simulink library "xbsIndex_r3"  (Simulink 6.1)
PreLoadFcn:
  | xlmeta;
undefined symbols (not defined in the file or in its folder): sim_pause
libraries: xbsIndex_r3 x62, simulink x1
(part 4 of 4)

== system xbsIndex_r3/ System Generator ==
  2x System Clock : DiscretePulseGenerator  SampleTime=simulink_period
  Continuous Source : DiscretePulseGenerator  PulseType=Time based  Period=2*simulink_period  PulseWidth=50
  Terminator : Terminator
  Terminator1 : Terminator
  wires:
  2x System Clock/1 -> Terminator/1
  Continuous Source/1 -> Terminator1/1

== system xbsIndex_r3/Configurable Subsystem Manager ==
  2x System Clock : DiscretePulseGenerator
  Continuous Source : DiscretePulseGenerator  PulseType=Time based  PulseWidth=50
  Terminator : Terminator
  Terminator1 : Terminator
  wires:
  2x System Clock/1 -> Terminator/1
  Continuous Source/1 -> Terminator1/1

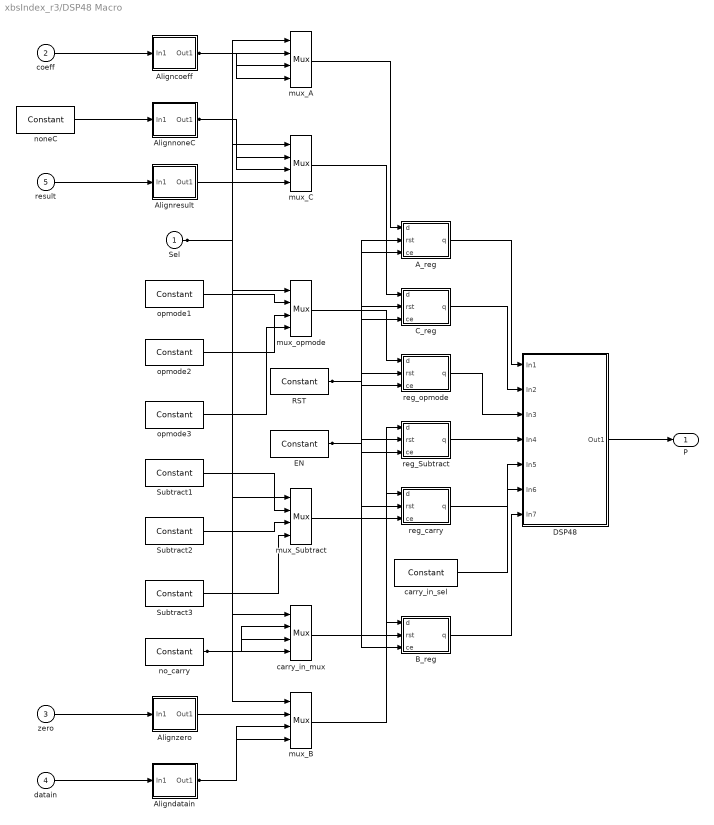
== system xbsIndex_r3/DSP48 Macro ==
  Sel : Inport  Port=1  LatchInput=off
  coeff : Inport  Port=2  LatchInput=off
  zero : Inport  Port=3  LatchInput=off
  datain : Inport  Port=4  LatchInput=off
  result : Inport  Port=5  LatchInput=off
  A_reg : Subsystem  mask{nreg=1, pnreg=1}
      mask prompts: nreg "Number of registers"; pnreg "Previous number of register"
      mask init:
      | [bg,fg] = xlcmap('XBlock',0);
      | iPos = get_param(gcb,'Position');
      | iWidth=iPos(3)-iPos(1); iHeight=iPos(4)-iPos(2);
      | iCx=iWidth/2;
      | iCy=iHeight/2;
      | [logoX, logoY] = xlogo(iPos);
      | str = sprintf('-%d',nreg);
      | sav_gcb = gcb;
      | set_param(sav_gcb,'linkstatus','none');
      | if (nreg ~= pnreg)
      |     sav_gcb  = gcb;
      |     regs     = find_system(sav_gcb, 'lookUnderMasks', 'all', 'masktype', 'Xilinx Register Block');
      |     terms    = find_system(sav_gcb, 'lookUnderMasks', 'all', 'BlockType', 'Terminator');
      |     inports  = find_system(sav_gcb, 'lookUnderMasks', 'all', 'BlockType', 'Inport');
      |     outports = find_system(sav_gcb, 'lookUnderMasks', 'all', 'BlockType', 'Outport');
      |       
      |     % delete all lines
      |     lines = get_param(sav_gcb, 'Lines');
      |     for i = 1:length(lines)
      |         delete_line(sav_gcb, lines(i,:).Points(1,:));
      |     end
      |       
      |     for i = 1:length(regs)
      |         delete_block(regs{i});
      |     end
      |     for i = 1:length(terms)
      |         delete_block(terms{i});
      |     end
      |     switch(nreg)
      |       case 0
      |           add_block('built-in/Terminator', [sav_gcb '/Terminator1'], 'position', [170   180   190   200]);
      |           add_block('built-in/Terminator', [sav_gcb '/Terminator2'], 'position', [240   195   260   215]);
      |           add_line(sav_gcb, 'd/1',   'q/1',           'autorouting', 'on');
      |           add_line(sav_gcb, 'rst/1', 'Terminator1/1', 'autorouting', 'on');
      |           add_line(sav_gcb, 'ce/1',  'Terminator2/1', 'autorouting', 'on');
      |       case 1
      |           add_block('xbsIndex_r3/Register', [sav_gcb '/Register1'], 'en', 'on', 'rst', 'on', 'position', [245   166   290   214]);
      |           add_line(sav_gcb, 'd/1',   'Register1/1',   'autorouting', 'on');
      |           add_line(sav_gcb, 'rst/1', 'Register1/2', 'autorouting', 'on');
      |           add_line(sav_gcb, 'ce/1',  'Register1/3', 'autorouting', 'on');
      |           add_line(sav_gcb, 'Register1/1', 'q/1',     'autorouting', 'on');
      |       case 2
      |           add_block('xbsIndex_r3/Register', [sav_gcb '/Register1'], 'en', 'on', 'rst', 'on', 'position', [245   166   290   214]);
      |           add_block('xbsIndex_r3/Register', [sav_gcb '/Register2'], 'en', 'on', 'rst', 'on', 'position', [385   181   430   229]);
      |           add_line(sav_gcb, 'd/1',   'Register1/1',   'autorouting', 'on');
      |           add_line(sav_gcb, 'rst/1', 'Register1/2', 'autorouting', 'on');
      |           add_line(sav_gcb, 'ce/1',  'Register1/3', 'autorouting', 'on');
      |           add_line(sav_gcb, 'Register1/1', 'Register2/1', 'autorouting', 'on');
      |           add_line(sav_gcb, 'rst/1', 'Register2/2', 'autorouting', 'on');
      |           add_line(sav_gcb, 'ce/1',  'Register2/3', 'autorouting', 'on');
      |           add_line(sav_gcb, 'Register2/1', 'q/1',   'autorouting', 'on');
      |      otherwise
      |           error('Illegal Mask Parameter to Register.  Allowed values are 0, 1, 2.');
      |     end
      |     set_param(sav_gcb, 'pnreg', int2str(nreg));
      | end
      mask Display:
      | patch([0 iWidth iWidth 0],[0 0 iHeight iHeight] , bg);
      | patch(logoX,logoY , fg);
      | text(iCx-6,iCy,'z');
      | text(iCx,iCy+4,str);
      | port_label('input',1,'d');
      | port_label('input',2,'rst');
      | port_label('input',3,'ce');
      | port_label('output',1,'q');
      | plot([0 0 iWidth iWidth 0], [0 iHeight iHeight 0 0]);
  Aligncoeff : Subsystem  mask{n_bits=18, bin_pt=11, arith_type=Signed  (2's comp), portwidth=18, dbl_ovrd=0}
      mask prompts: n_bits "Number of bits"; bin_pt "Binary Point"; arith_type "Arithmetic type"; portwidth "Port width"
      mask init:
      | this_gcb = gcb;
      | set_param(this_gcb,'linkstatus','none');
      | [bg,fg] = xlcmap('XBlock',dbl_ovrd);
      | iPos = get_param(gcb,'Position');
      | iWidth=iPos(3)-iPos(1); iHeight=iPos(4)-iPos(2);
      | iCx=iWidth/2;
      | iCy=iHeight/2;
      | [logoX, logoY] = xlogo(iPos);
      mask StyleString: edit,edit,popup(Signed  (2's comp)|Unsigned),edit,edit
      mask Display:
      | patch([0 iWidth iWidth 0],[0 0 iHeight iHeight] , bg);
      | patch(logoX,logoY , fg);
      | plot([0 0 iWidth iWidth 0], [0 iHeight iHeight 0 0]);
  Aligndatain : Subsystem  mask{n_bits=18, bin_pt=0, arith_type=Signed  (2's comp), portwidth=18, dbl_ovrd=0}
      mask prompts: n_bits "Number of bits"; bin_pt "Binary Point"; arith_type "Arithmetic type"; portwidth "Port width"
      mask init: same as xbsIndex_r3/DSP48 Macro/Aligncoeff
      mask StyleString: edit,edit,popup(Signed  (2's comp)|Unsigned),edit,edit
      mask Display:
      | patch([0 iWidth iWidth 0],[0 0 iHeight iHeight] , bg);
      | patch(logoX,logoY , fg);
      | plot([0 0 iWidth iWidth 0], [0 iHeight iHeight 0 0]);
  AlignnoneC : Subsystem  mask{n_bits=48, bin_pt=0, arith_type=Signed  (2's comp), portwidth=48, dbl_ovrd=0}
      mask prompts: n_bits "Number of bits"; bin_pt "Binary Point"; arith_type "Arithmetic type"; portwidth "Port width"
      mask init: same as xbsIndex_r3/DSP48 Macro/Aligncoeff
      mask StyleString: edit,edit,popup(Signed  (2's comp)|Unsigned),edit,edit
      mask Display:
      | patch([0 iWidth iWidth 0],[0 0 iHeight iHeight] , bg);
      | patch(logoX,logoY , fg);
      | plot([0 0 iWidth iWidth 0], [0 iHeight iHeight 0 0]);
  Alignresult : Subsystem  mask{n_bits=41, bin_pt=11, arith_type=Signed  (2's comp), portwidth=48, dbl_ovrd=0}
      mask prompts: n_bits "Number of bits"; bin_pt "Binary Point"; arith_type "Arithmetic type"; portwidth "Port width"
      mask init: same as xbsIndex_r3/DSP48 Macro/Aligncoeff
      mask StyleString: edit,edit,popup(Signed  (2's comp)|Unsigned),edit,edit
      mask Display:
      | patch([0 iWidth iWidth 0],[0 0 iHeight iHeight] , bg);
      | patch(logoX,logoY , fg);
      | plot([0 0 iWidth iWidth 0], [0 iHeight iHeight 0 0]);
  Alignzero : Subsystem  mask{n_bits=18, bin_pt=0, arith_type=Signed  (2's comp), portwidth=18, dbl_ovrd=0}
      mask prompts: n_bits "Number of bits"; bin_pt "Binary Point"; arith_type "Arithmetic type"; portwidth "Port width"
      mask init: same as xbsIndex_r3/DSP48 Macro/Aligncoeff
      mask StyleString: edit,edit,popup(Signed  (2's comp)|Unsigned),edit,edit
      mask Display:
      | patch([0 iWidth iWidth 0],[0 0 iHeight iHeight] , bg);
      | patch(logoX,logoY , fg);
      | plot([0 0 iWidth iWidth 0], [0 iHeight iHeight 0 0]);
  B_reg : Subsystem  mask{nreg=1, pnreg=1}
      mask prompts: nreg "Number of registers"; pnreg "Previous number of register"
      mask init: same as xbsIndex_r3/DSP48 Macro/A_reg
      mask Display:
      | patch([0 iWidth iWidth 0],[0 0 iHeight iHeight] , bg);
      | patch(logoX,logoY , fg);
      | text(iCx-6,iCy,'z');
      | text(iCx,iCy+4,str);
      | port_label('input',1,'d');
      | port_label('input',2,'rst');
      | port_label('input',3,'ce');
      | port_label('output',1,'q');
      | plot([0 0 iWidth iWidth 0], [0 iHeight iHeight 0 0]);
  C_reg : Subsystem  mask{nreg=2, pnreg=2}
      mask prompts: nreg "Number of registers"; pnreg "Previous number of register"
      mask init: same as xbsIndex_r3/DSP48 Macro/A_reg
      mask Display:
      | patch([0 iWidth iWidth 0],[0 0 iHeight iHeight] , bg);
      | patch(logoX,logoY , fg);
      | text(iCx-6,iCy,'z');
      | text(iCx,iCy+4,str);
      | port_label('input',1,'d');
      | port_label('input',2,'rst');
      | port_label('input',3,'ce');
      | port_label('output',1,'q');
      | plot([0 0 iWidth iWidth 0], [0 iHeight iHeight 0 0]);
  DSP48 : Subsystem  mask{dbl_ovrd=0}
      mask init:
      | this_gcb = gcb;
      | [bg,fg] = xlcmap('XBlock',dbl_ovrd);
      | iPos = get_param(gcb,'Position');
      | iWidth=iPos(3)-iPos(1); iHeight=iPos(4)-iPos(2);
      | iCx=iWidth/2;
      | iCy=iHeight/2;
      | [logoX, logoY] = xlogo(iPos);
      | set_param(this_gcb,'linkstatus','none');
      mask Display:
      | patch([0 iWidth iWidth 0],[0 0 iHeight iHeight] , bg);
      | patch(logoX,logoY , fg);
      | plot([0 0 iWidth iWidth 0], [0 iHeight iHeight 0 0]);
      | port_label('input',1,'A');
      | port_label('input',2,'C');
      | port_label('input',3,'Opmode');
      | port_label('input',4,'Subtract_sel');
      | port_label('input',5,'Carry');
      | port_label('input',6,'Carry_in_sel');
      | port_label('input',7,'B');
      | port_label('output',1,'P');
  EN : xbsIndex_r3/Constant  const=1  equ=P=C  arith_type=Boolean  n_bits=1  bin_pt=0  opselect=C  inp2=PCIN>>17  opr=+  inp1=P  carry=CIN  iostate=0  explicit_period=off  period=1  dbl_ovrd=off
  RST : xbsIndex_r3/Constant  const=0  equ=P=C  arith_type=Boolean  n_bits=1  bin_pt=0  opselect=C  inp2=PCIN>>17  opr=+  inp1=P  carry=CIN  iostate=0  explicit_period=off  period=1  dbl_ovrd=off
  Subtract1 : xbsIndex_r3/Constant  Tag=1  const=0  equ=P=C  arith_type=Boolean  n_bits=1  bin_pt=0  opselect=C  inp2=PCIN>>17  opr=+  inp1=P  carry=CIN  iostate=0  explicit_period=off  period=1  dbl_ovrd=off
  Subtract2 : xbsIndex_r3/Constant  Tag=2  const=0  equ=P=C  arith_type=Boolean  n_bits=1  bin_pt=0  opselect=C  inp2=PCIN>>17  opr=+  inp1=P  carry=CIN  iostate=0  explicit_period=off  period=1  dbl_ovrd=off
  Subtract3 : xbsIndex_r3/Constant  Tag=3  const=0  equ=P=C  arith_type=Boolean  n_bits=1  bin_pt=0  opselect=C  inp2=PCIN>>17  opr=+  inp1=P  carry=CIN  iostate=0  explicit_period=off  period=1  dbl_ovrd=off
  carry_in_mux : xbsIndex_r3/Mux  inputs=3  precision=Full  arith_type="Signed  (2's comp)"  n_bits=8  bin_pt=2  quantization=Truncate  overflow=Wrap  latency=0  explicit_period=off  period=1  en=off  dbl_ovrd=off  show_param=off  mux_type=off  use_rpm=off  gen_core=off
      settings: xl_area=[0, 0, 0, 0, 0, 0, 0]
  carry_in_sel : xbsIndex_r3/Constant  const=0  equ=P=C  arith_type=Unsigned  n_bits=2  bin_pt=0  opselect=C  inp2=PCIN>>17  opr=+  inp1=P  carry=CIN  iostate=0  explicit_period=off  period=1  dbl_ovrd=off
  mux_A : xbsIndex_r3/Mux  inputs=3  precision=User Defined  arith_type="Signed  (2's comp)"  n_bits=18  bin_pt=0  quantization=Truncate  overflow=Wrap  latency=0  explicit_period=off  period=1  en=off  dbl_ovrd=off  show_param=off  mux_type=off  use_rpm=off  gen_core=off
      settings: xl_area=[0, 0, 0, 0, 0, 0, 0]
  mux_B : xbsIndex_r3/Mux  inputs=3  precision=User Defined  arith_type="Signed  (2's comp)"  n_bits=18  bin_pt=0  quantization=Truncate  overflow=Wrap  latency=0  explicit_period=off  period=1  en=off  dbl_ovrd=off  show_param=off  mux_type=off  use_rpm=off  gen_core=off
      settings: xl_area=[0, 0, 0, 0, 0, 0, 0]
  mux_C : xbsIndex_r3/Mux  inputs=3  precision=User Defined  arith_type="Signed  (2's comp)"  n_bits=48  bin_pt=0  quantization=Truncate  overflow=Wrap  latency=0  explicit_period=off  period=1  en=off  dbl_ovrd=off  show_param=off  mux_type=off  use_rpm=off  gen_core=off
      settings: xl_area=[0, 0, 0, 0, 0, 0, 0]
  mux_Subtract : xbsIndex_r3/Mux  inputs=3  precision=Full  arith_type="Signed  (2's comp)"  n_bits=8  bin_pt=2  quantization=Truncate  overflow=Wrap  latency=0  explicit_period=off  period=1  en=off  dbl_ovrd=off  show_param=off  mux_type=off  use_rpm=off  gen_core=off
      settings: xl_area=[0, 0, 0, 0, 0, 0, 0]
  mux_opmode : xbsIndex_r3/Mux  inputs=3  precision=Full  arith_type="Signed  (2's comp)"  n_bits=8  bin_pt=2  quantization=Truncate  overflow=Wrap  latency=0  explicit_period=off  period=1  en=off  dbl_ovrd=off  show_param=off  mux_type=off  use_rpm=off  gen_core=off
      settings: xl_area=[0, 0, 0, 0, 0, 0, 0]
  no_carry : xbsIndex_r3/Constant  const=0  equ=P=C  arith_type=Unsigned  n_bits=1  bin_pt=0  opselect=C  inp2=PCIN>>17  opr=+  inp1=P  carry=CIN  iostate=0  explicit_period=off  period=1  dbl_ovrd=off
  noneC : xbsIndex_r3/Constant  const=0  equ=P=C  arith_type=Unsigned  n_bits=1  bin_pt=0  opselect=C  inp2=PCIN>>17  opr=+  inp1=P  carry=CIN  iostate=0  explicit_period=off  period=1  dbl_ovrd=off
  opmode1 : xbsIndex_r3/Constant  Tag=1  const=37  equ=P=C  arith_type=Unsigned  n_bits=7  bin_pt=0  opselect=C  inp2=PCIN>>17  opr=+  inp1=P  carry=CIN  iostate=0  explicit_period=off  period=1  dbl_ovrd=off
  opmode2 : xbsIndex_r3/Constant  Tag=2  const=5  equ=P=C  arith_type=Unsigned  n_bits=7  bin_pt=0  opselect=C  inp2=PCIN>>17  opr=+  inp1=P  carry=CIN  iostate=0  explicit_period=off  period=1  dbl_ovrd=off
  opmode3 : xbsIndex_r3/Constant  Tag=3  const=53  equ=P=C  arith_type=Unsigned  n_bits=7  bin_pt=0  opselect=C  inp2=PCIN>>17  opr=+  inp1=P  carry=CIN  iostate=0  explicit_period=off  period=1  dbl_ovrd=off
  reg_Subtract : Subsystem  mask{nreg=2, pnreg=2}
      mask prompts: nreg "Number of registers"; pnreg "Previous number of register"
      mask init: same as xbsIndex_r3/DSP48 Macro/A_reg
      mask Display:
      | patch([0 iWidth iWidth 0],[0 0 iHeight iHeight] , bg);
      | patch(logoX,logoY , fg);
      | text(iCx-6,iCy,'z');
      | text(iCx,iCy+4,str);
      | port_label('input',1,'d');
      | port_label('input',2,'rst');
      | port_label('input',3,'ce');
      | port_label('output',1,'q');
      | plot([0 0 iWidth iWidth 0], [0 iHeight iHeight 0 0]);
  reg_carry : Subsystem  mask{nreg=2, pnreg=2}
      mask prompts: nreg "Number of registers"; pnreg "Previous number of register"
      mask init: same as xbsIndex_r3/DSP48 Macro/A_reg
      mask Display:
      | patch([0 iWidth iWidth 0],[0 0 iHeight iHeight] , bg);
      | patch(logoX,logoY , fg);
      | text(iCx-6,iCy,'z');
      | text(iCx,iCy+4,str);
      | port_label('input',1,'d');
      | port_label('input',2,'rst');
      | port_label('input',3,'ce');
      | port_label('output',1,'q');
      | plot([0 0 iWidth iWidth 0], [0 iHeight iHeight 0 0]);
  reg_opmode : Subsystem  mask{nreg=2, pnreg=2}
      mask prompts: nreg "Number of registers"; pnreg "Previous number of register"
      mask init: same as xbsIndex_r3/DSP48 Macro/A_reg
      mask Display:
      | patch([0 iWidth iWidth 0],[0 0 iHeight iHeight] , bg);
      | patch(logoX,logoY , fg);
      | text(iCx-6,iCy,'z');
      | text(iCx,iCy+4,str);
      | port_label('input',1,'d');
      | port_label('input',2,'rst');
      | port_label('input',3,'ce');
      | port_label('output',1,'q');
      | plot([0 0 iWidth iWidth 0], [0 iHeight iHeight 0 0]);
  P : Outport
  wires:
  Sel/1 -> mux_C/1, mux_B/1, mux_A/1, carry_in_mux/1, mux_Subtract/1, mux_opmode/1
  RST/1 -> C_reg/2(rst), B_reg/2(rst), A_reg/2(rst), reg_carry/2(rst), reg_Subtract/2(rst), reg_opmode/2(rst)
  EN/1 -> C_reg/3(ce), B_reg/3(ce), A_reg/3(ce), reg_carry/3(ce), reg_Subtract/3(ce), reg_opmode/3(ce)
  no_carry/1 -> carry_in_mux/4, carry_in_mux/3, carry_in_mux/2
  Aligncoeff/1(Out1) -> mux_A/4, mux_A/3, mux_A/2
  Aligndatain/1(Out1) -> mux_B/4, mux_B/3
  AlignnoneC/1(Out1) -> mux_C/3, mux_C/2
  Alignresult/1(Out1) -> mux_C/4
  result/1 -> Alignresult/1(In1)
  noneC/1 -> AlignnoneC/1(In1)
  C_reg/1(q) -> DSP48/2(In2)
  mux_C/1 -> C_reg/1(d)
  datain/1 -> Aligndatain/1(In1)
  Alignzero/1(Out1) -> mux_B/2
  zero/1 -> Alignzero/1(In1)
  B_reg/1(q) -> DSP48/7(In7)
  mux_B/1 -> B_reg/1(d)
  coeff/1 -> Aligncoeff/1(In1)
  A_reg/1(q) -> DSP48/1(In1)
  mux_A/1 -> A_reg/1(d)
  reg_carry/1(q) -> DSP48/5(In5)
  carry_in_mux/1 -> reg_carry/1(d)
  carry_in_sel/1 -> DSP48/6(In6)
  Subtract3/1 -> mux_Subtract/4
  Subtract2/1 -> mux_Subtract/3
  Subtract1/1 -> mux_Subtract/2
  reg_Subtract/1(q) -> DSP48/4(In4)
  mux_Subtract/1 -> reg_Subtract/1(d)
  opmode3/1 -> mux_opmode/4
  opmode2/1 -> mux_opmode/3
  opmode1/1 -> mux_opmode/2
  reg_opmode/1(q) -> DSP48/3(In3)
  mux_opmode/1 -> reg_opmode/1(d)
  DSP48/1(Out1) -> P/1

== system xbsIndex_r3/Disregard Subsystem ==

== system xbsIndex_r3/FDATool ==
  Constant : Constant  Value=0  VectorParams1D=off  OutDataTypeMode=double
  Terminator : Terminator
  wires:
  Constant/1 -> Terminator/1

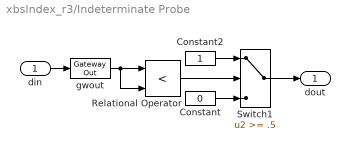
== system xbsIndex_r3/Indeterminate Probe ==
  din : Inport  Port=1  LatchInput=off
  Constant : Constant  Value=0
  Constant2 : Constant
  Relational Operator : RelationalOperator  Operator=<  InputSameDT=on
  Switch1 : Switch  Threshold=.5  SaturateOnIntegerOverflow=on  InputSameDT=on
  gwout : xbsIndex_r3/Gateway Out  output_type=Double  nbits=8  bin_pt=6  arith_type=Boolean  quantization=Truncate  overflow=Wrap  hdl_port=off  timing_constraint=None  locs_specified=off  LOCs={}  needs_fixed_name=off  show_param=off
      settings: xl_area=[0, 0, 0, 0, 0, 0, 0]
  dout : Outport
  wires:
  Switch1/1 -> dout/1
  Constant/1 -> Switch1/3
  Constant2/1 -> Switch1/1
  gwout/1 -> Relational Operator/2, Relational Operator/1
  Relational Operator/1 -> Switch1/2
  din/1 -> gwout/1

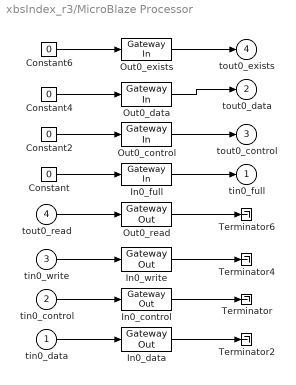
== system xbsIndex_r3/MicroBlaze Processor ==
  tin0_data : Inport  Tag=in0  Port=1  LatchInput=off
  tin0_control : Inport  Tag=in0  Port=2  LatchInput=off
  tin0_write : Inport  Tag=in0  Port=3  LatchInput=off
  tout0_read : Inport  Tag=out0  Port=4  LatchInput=off
  Constant{,2,4,6} (4 alike) : Constant  Value=0
  In0_control : xbsIndex_r3/Gateway Out  output_type=Double  nbits=8  bin_pt=6  arith_type=Boolean  quantization=Truncate  overflow=Wrap  hdl_port=on  timing_constraint=None  locs_specified=off  LOCs={}  needs_fixed_name=off  show_param=off
      settings: xl_area=[0, 0, 0, 0, 0, 0, 0]
  In0_data : xbsIndex_r3/Gateway Out  output_type=Double  nbits=8  bin_pt=6  arith_type=Boolean  quantization=Truncate  overflow=Wrap  hdl_port=on  timing_constraint=None  locs_specified=off  LOCs={}  needs_fixed_name=off  show_param=off
      settings: xl_area=[0, 0, 0, 0, 0, 0, 0]
  In0_full : xbsIndex_r3/Gateway In  arith_type=Unsigned  n_bits=1  bin_pt=0  quantization=Truncate  overflow=Wrap  period=1  timing_constraint=None  locs_specified=off  LOCs={}  needs_fixed_name=off  dbl_ovrd=off  show_param=off
      settings: xl_area=[0, 0, 0, 0, 0, 0, 0]
  In0_write : xbsIndex_r3/Gateway Out  output_type=Double  nbits=8  bin_pt=6  arith_type=Boolean  quantization=Truncate  overflow=Wrap  hdl_port=on  timing_constraint=None  locs_specified=off  LOCs={}  needs_fixed_name=off  show_param=off
      settings: xl_area=[0, 0, 0, 0, 0, 0, 0]
  Out0_control : xbsIndex_r3/Gateway In  arith_type=Unsigned  n_bits=1  bin_pt=0  quantization=Truncate  overflow=Wrap  period=1  timing_constraint=None  locs_specified=off  LOCs={}  needs_fixed_name=off  dbl_ovrd=off  show_param=off
      settings: xl_area=[0, 0, 0, 0, 0, 0, 0]
  Out0_data : xbsIndex_r3/Gateway In  arith_type=Unsigned  n_bits=32  bin_pt=0  quantization=Truncate  overflow=Wrap  period=1  timing_constraint=None  locs_specified=off  LOCs={}  needs_fixed_name=off  dbl_ovrd=off  show_param=off
      settings: xl_area=[0, 0, 0, 0, 0, 0, 0]
  Out0_exists : xbsIndex_r3/Gateway In  arith_type=Unsigned  n_bits=1  bin_pt=0  quantization=Truncate  overflow=Wrap  period=1  timing_constraint=None  locs_specified=off  LOCs={}  needs_fixed_name=off  dbl_ovrd=off  show_param=off
      settings: xl_area=[0, 0, 0, 0, 0, 0, 0]
  Out0_read : xbsIndex_r3/Gateway Out  output_type=Double  nbits=8  bin_pt=6  arith_type=Boolean  quantization=Truncate  overflow=Wrap  hdl_port=on  timing_constraint=None  locs_specified=off  LOCs={}  needs_fixed_name=off  show_param=off
      settings: xl_area=[0, 0, 0, 0, 0, 0, 0]
  Terminator{,2,4,6} (4 alike) : Terminator
  tin0_full : Outport  Tag=in0
  tout0_data : Outport  Tag=out0  Port=2
  tout0_control : Outport  Tag=out0  Port=3
  tout0_exists : Outport  Tag=out0  Port=4
  wires:
  Out0_read/1 -> Terminator6/1
  Constant6/1 -> Out0_exists/1
  Constant4/1 -> Out0_data/1
  Constant2/1 -> Out0_control/1
  In0_write/1 -> Terminator4/1
  Constant/1 -> In0_full/1
  In0_data/1 -> Terminator2/1
  In0_control/1 -> Terminator/1
  Out0_exists/1 -> tout0_exists/1
  Out0_control/1 -> tout0_control/1
  Out0_data/1 -> tout0_data/1
  In0_full/1 -> tin0_full/1
  tout0_read/1 -> Out0_read/1
  tin0_write/1 -> In0_write/1
  tin0_control/1 -> In0_control/1
  tin0_data/1 -> In0_data/1

== system xbsIndex_r3/Multiple Subsystem Generator ==
  note: This is the Design Stitcher tool.
  Constant : Constant
  Terminator : Terminator
  wires:
  Constant/1 -> Terminator/1

== system xbsIndex_r3/Pause Simulation ==
  din : Inport  Port=1  LatchInput=off
  Gateway Out : xbsIndex_r3/Gateway Out  output_type=Double  nbits=8  bin_pt=6  arith_type=Boolean  quantization=Truncate  overflow=Wrap  hdl_port=on  timing_constraint=None  locs_specified=off  LOCs={}  needs_fixed_name=off  show_param=off
      settings: xl_area=[0, 0, 0, 0, 0, 0, 0]
  Pause  Simulation : MATLABFcn  Priority=1000  MATLABFcn=sim_pause(u)  OutputDimensions=0  Output1D=off
  wires:
  din/1 -> Gateway Out/1
  Gateway Out/1 -> Pause  Simulation/1

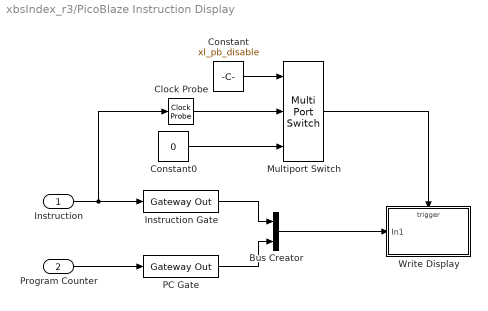
== system xbsIndex_r3/PicoBlaze Instruction Display ==
  Instruction : Inport  Port=1  LatchInput=off
  Program Counter : Inport  Port=2  LatchInput=off
  Bus Creator : BusCreator  DialogController=Simulink.DDGSource_Bus  Inputs=2
  Clock Probe : xbsIndex_r3/Clock Probe
  Constant : Constant  Value=xl_pb_disable
  Constant0 : Constant  Value=0
  Instruction Gate : xbsIndex_r3/Gateway Out  output_type=Double  nbits=8  bin_pt=6  arith_type=Boolean  quantization=Truncate  overflow=Wrap  hdl_port=off  timing_constraint=None  locs_specified=off  LOCs={}  needs_fixed_name=off  show_param=off
      settings: xl_area=[0, 0, 0, 0, 0, 0, 0]
  Multiport Switch : MultiPortSwitch  Inputs=2  zeroidx=on  SaturateOnIntegerOverflow=on
  PC Gate : xbsIndex_r3/Gateway Out  output_type=Double  nbits=8  bin_pt=6  arith_type=Boolean  quantization=Truncate  overflow=Wrap  hdl_port=off  timing_constraint=None  locs_specified=off  LOCs={}  needs_fixed_name=off  show_param=off
      settings: xl_area=[0, 0, 0, 0, 0, 0, 0]
  Write Display : Subsystem  mask{xl_pb_inst=LOAD sC, 12, xl_pb_pc=17, xl_pb_version=xl_pb_version}
      mask prompts: xl_pb_version "PicoBlaze Version"
  wires:
  Bus Creator/1 -> Write Display/1(In1)
  PC Gate/1 -> Bus Creator/2
  Instruction Gate/1 -> Bus Creator/1
  Program Counter/1 -> PC Gate/1
  Instruction/1 -> Instruction Gate/1, Clock Probe/1
  Constant/1 -> Multiport Switch/1
  Multiport Switch/1 -> Write Display/Trigger
  Clock Probe/1 -> Multiport Switch/2
  Constant0/1 -> Multiport Switch/3

== system xbsIndex_r3/Resource Estimator ==
  2x System Clock : DiscretePulseGenerator  SampleTime=simulink_period
  Terminator : Terminator
  wires:
  2x System Clock/1 -> Terminator/1

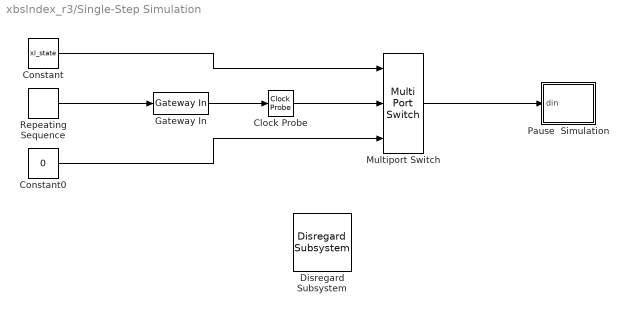
== system xbsIndex_r3/Single-Step Simulation ==
  Clock Probe : xbsIndex_r3/Clock Probe
  Constant : Constant  Value=xl_state
  Constant0 : Constant  Value=0
  Disregard Subsystem : xbsIndex_r3/Disregard Subsystem  Tag=discardX
      settings: AttributesFormatString=Disregard Subsystem\nFor Generation
  Gateway In : xbsIndex_r3/Gateway In  arith_type=Boolean  n_bits=8  bin_pt=6  quantization=Truncate  overflow=Wrap  period=1  timing_constraint=None  locs_specified=off  LOCs={}  needs_fixed_name=off  dbl_ovrd=off  show_param=off
      settings: xl_area=[0, 0, 0, 0, 0, 0, 0]
  Multiport Switch : MultiPortSwitch  Inputs=2  zeroidx=on  SaturateOnIntegerOverflow=on
  Pause  Simulation : Subsystem  mask(Xilinx Pause Simulation.){}
      mask help: Pause Simulation. Pause simulation when the input is non-zero.
      mask init:
      | [bg,fg] = xlcmap('XTool',0);
      | iPos = get_param(gcb,'Position');
      | iWidth=iPos(3)-iPos(1); iHeight=iPos(4)-iPos(2);
      | iCx=iWidth/2;
      | iCy=iHeight/2;
      | [logoX, logoY] = xlogo(iPos);
      mask Display:
      | patch([0 iWidth iWidth 0],[0 0 iHeight iHeight] , bg);
      | patch(logoX,logoY , fg);
      | ;plot([0 0 iWidth iWidth 0], [0 iHeight iHeight 0 0]);
  Repeating Sequence : simulink/Sources/Repeating Sequence  rep_seq_t=[0 1]  rep_seq_y=[1 1]
  wires:
  Gateway In/1 -> Clock Probe/1
  Repeating Sequence/1 -> Gateway In/1
  Multiport Switch/1 -> Pause  Simulation/1(din)
  Clock Probe/1 -> Multiport Switch/2
  Constant0/1 -> Multiport Switch/3
  Constant/1 -> Multiport Switch/1

== system xbsIndex_r3/Toolbar ==
  note: This is the toolbar tool.
  Constant : Constant
  Terminator : Terminator
  wires:
  Constant/1 -> Terminator/1

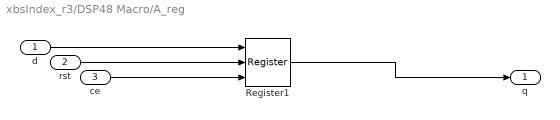
== system xbsIndex_r3/DSP48 Macro/A_reg ==
  d : Inport  Port=1  LatchInput=off
  rst : Inport  Port=2  LatchInput=off
  ce : Inport  Port=3  LatchInput=off
  Register1 : xbsIndex_r3/Register  init=0  reg_only_valid=off  explicit_period=off  period=1  rst=on  en=on  out_en=off  dbl_ovrd=off  show_param=off
      settings: xl_area=[0, 0, 0, 0, 0, 0, 0]
  q : Outport
  wires:
  Register1/1 -> q/1
  ce/1 -> Register1/3
  rst/1 -> Register1/2
  d/1 -> Register1/1

== system xbsIndex_r3/DSP48 Macro/Aligncoeff ==
  In1 : Inport  Port=1  LatchInput=off
  Align : xbsIndex_r3/Convert  arith_type="Signed  (2's comp)"  n_bits=n_bits  bin_pt=bin_pt  quantization=Truncate  overflow=Wrap  latency=0  explicit_period=off  period=1  dbl_ovrd=off  show_param=off  inserted_by_tool=off  pipeline=off
      settings: xl_area=[0, 0, 0, 0, 0, 0, 0]
  Prec : xbsIndex_r3/Convert  arith_type="Signed  (2's comp)"  n_bits=portwidth  bin_pt=0  quantization=Truncate  overflow=Wrap  latency=0  explicit_period=off  period=1  dbl_ovrd=off  show_param=off  inserted_by_tool=off  pipeline=off
      settings: xl_area=[0, 0, 0, 0, 0, 0, 0]
  Reinterpret : xbsIndex_r3/Reinterpret  force_arith_type=off  arith_type=Unsigned  force_bin_pt=on  bin_pt=0  force_valid=on
  Out1 : Outport
  wires:
  Prec/1 -> Out1/1
  In1/1 -> Align/1
  Reinterpret/1 -> Prec/1
  Align/1 -> Reinterpret/1

== system xbsIndex_r3/DSP48 Macro/Aligndatain ==
  In1 : Inport  Port=1  LatchInput=off
  Align : xbsIndex_r3/Convert  arith_type="Signed  (2's comp)"  n_bits=n_bits  bin_pt=bin_pt  quantization=Truncate  overflow=Wrap  latency=0  explicit_period=off  period=1  dbl_ovrd=off  show_param=off  inserted_by_tool=off  pipeline=off
      settings: xl_area=[0, 0, 0, 0, 0, 0, 0]
  Prec : xbsIndex_r3/Convert  arith_type="Signed  (2's comp)"  n_bits=portwidth  bin_pt=0  quantization=Truncate  overflow=Wrap  latency=0  explicit_period=off  period=1  dbl_ovrd=off  show_param=off  inserted_by_tool=off  pipeline=off
      settings: xl_area=[0, 0, 0, 0, 0, 0, 0]
  Reinterpret : xbsIndex_r3/Reinterpret  force_arith_type=off  arith_type=Unsigned  force_bin_pt=on  bin_pt=0  force_valid=on
  Out1 : Outport
  wires:
  Prec/1 -> Out1/1
  In1/1 -> Align/1
  Reinterpret/1 -> Prec/1
  Align/1 -> Reinterpret/1

== system xbsIndex_r3/DSP48 Macro/AlignnoneC ==
  In1 : Inport  Port=1  LatchInput=off
  Align : xbsIndex_r3/Convert  arith_type="Signed  (2's comp)"  n_bits=n_bits  bin_pt=bin_pt  quantization=Truncate  overflow=Wrap  latency=0  explicit_period=off  period=1  dbl_ovrd=off  show_param=off  inserted_by_tool=off  pipeline=off
      settings: xl_area=[0, 0, 0, 0, 0, 0, 0]
  Prec : xbsIndex_r3/Convert  arith_type="Signed  (2's comp)"  n_bits=portwidth  bin_pt=0  quantization=Truncate  overflow=Wrap  latency=0  explicit_period=off  period=1  dbl_ovrd=off  show_param=off  inserted_by_tool=off  pipeline=off
      settings: xl_area=[0, 0, 0, 0, 0, 0, 0]
  Reinterpret : xbsIndex_r3/Reinterpret  force_arith_type=off  arith_type=Unsigned  force_bin_pt=on  bin_pt=0  force_valid=on
  Out1 : Outport
  wires:
  Prec/1 -> Out1/1
  In1/1 -> Align/1
  Reinterpret/1 -> Prec/1
  Align/1 -> Reinterpret/1

== system xbsIndex_r3/DSP48 Macro/Alignresult ==
  In1 : Inport  Port=1  LatchInput=off
  Align : xbsIndex_r3/Convert  arith_type="Signed  (2's comp)"  n_bits=n_bits  bin_pt=bin_pt  quantization=Truncate  overflow=Wrap  latency=0  explicit_period=off  period=1  dbl_ovrd=off  show_param=off  inserted_by_tool=off  pipeline=off
      settings: xl_area=[0, 0, 0, 0, 0, 0, 0]
  Prec : xbsIndex_r3/Convert  arith_type="Signed  (2's comp)"  n_bits=portwidth  bin_pt=0  quantization=Truncate  overflow=Wrap  latency=0  explicit_period=off  period=1  dbl_ovrd=off  show_param=off  inserted_by_tool=off  pipeline=off
      settings: xl_area=[0, 0, 0, 0, 0, 0, 0]
  Reinterpret : xbsIndex_r3/Reinterpret  force_arith_type=off  arith_type=Unsigned  force_bin_pt=on  bin_pt=0  force_valid=on
  Out1 : Outport
  wires:
  Prec/1 -> Out1/1
  In1/1 -> Align/1
  Reinterpret/1 -> Prec/1
  Align/1 -> Reinterpret/1

== system xbsIndex_r3/DSP48 Macro/Alignzero ==
  In1 : Inport  Port=1  LatchInput=off
  Align : xbsIndex_r3/Convert  arith_type="Signed  (2's comp)"  n_bits=n_bits  bin_pt=bin_pt  quantization=Truncate  overflow=Wrap  latency=0  explicit_period=off  period=1  dbl_ovrd=off  show_param=off  inserted_by_tool=off  pipeline=off
      settings: xl_area=[0, 0, 0, 0, 0, 0, 0]
  Prec : xbsIndex_r3/Convert  arith_type="Signed  (2's comp)"  n_bits=portwidth  bin_pt=0  quantization=Truncate  overflow=Wrap  latency=0  explicit_period=off  period=1  dbl_ovrd=off  show_param=off  inserted_by_tool=off  pipeline=off
      settings: xl_area=[0, 0, 0, 0, 0, 0, 0]
  Reinterpret : xbsIndex_r3/Reinterpret  force_arith_type=off  arith_type=Unsigned  force_bin_pt=on  bin_pt=0  force_valid=on
  Out1 : Outport
  wires:
  Prec/1 -> Out1/1
  In1/1 -> Align/1
  Reinterpret/1 -> Prec/1
  Align/1 -> Reinterpret/1

== system xbsIndex_r3/DSP48 Macro/B_reg ==
  d : Inport  Port=1  LatchInput=off
  rst : Inport  Port=2  LatchInput=off
  ce : Inport  Port=3  LatchInput=off
  Register1 : xbsIndex_r3/Register  init=0  reg_only_valid=off  explicit_period=off  period=1  rst=on  en=on  out_en=off  dbl_ovrd=off  show_param=off
      settings: xl_area=[0, 0, 0, 0, 0, 0, 0]
  q : Outport
  wires:
  Register1/1 -> q/1
  ce/1 -> Register1/3
  rst/1 -> Register1/2
  d/1 -> Register1/1

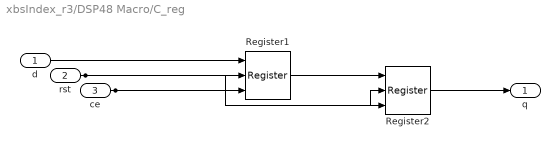
== system xbsIndex_r3/DSP48 Macro/C_reg ==
  d : Inport  Port=1  LatchInput=off
  rst : Inport  Port=2  LatchInput=off
  ce : Inport  Port=3  LatchInput=off
  Register1 : xbsIndex_r3/Register  init=0  reg_only_valid=off  explicit_period=off  period=1  rst=on  en=on  out_en=off  dbl_ovrd=off  show_param=off
      settings: xl_area=[0, 0, 0, 0, 0, 0, 0]
  Register2 : xbsIndex_r3/Register  init=0  reg_only_valid=off  explicit_period=off  period=1  rst=on  en=on  out_en=off  dbl_ovrd=off  show_param=off
      settings: xl_area=[0, 0, 0, 0, 0, 0, 0]
  q : Outport
  wires:
  d/1 -> Register1/1
  rst/1 -> Register1/2, Register2/2
  ce/1 -> Register1/3, Register2/3
  Register1/1 -> Register2/1
  Register2/1 -> q/1

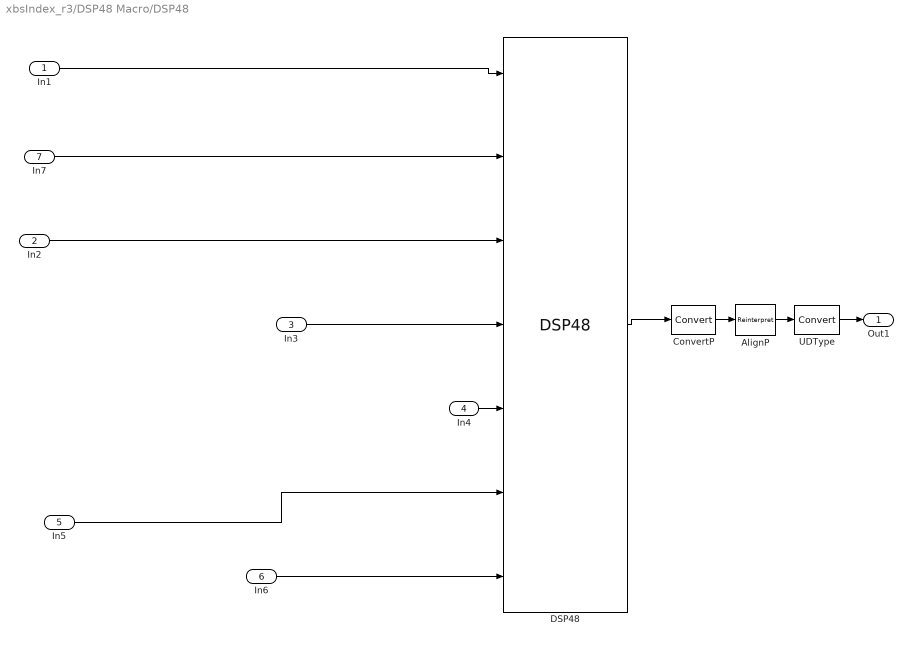
== system xbsIndex_r3/DSP48 Macro/DSP48 ==
  In1 : Inport  Port=1  LatchInput=off
  In2 : Inport  Port=2  LatchInput=off
  In3 : Inport  Port=3  LatchInput=off
  In4 : Inport  Port=4  LatchInput=off
  In5 : Inport  Port=5  LatchInput=off
  In6 : Inport  Port=6  LatchInput=off
  In7 : Inport  Port=7  LatchInput=off
  AlignP : xbsIndex_r3/Reinterpret  force_arith_type=on  arith_type=Unsigned  force_bin_pt=on  bin_pt=11  force_valid=on
  ConvertP : xbsIndex_r3/Convert  arith_type="Signed  (2's comp)"  n_bits=48  bin_pt=0  quantization=Truncate  overflow=Wrap  latency=0  explicit_period=off  period=1  dbl_ovrd=off  show_param=off  inserted_by_tool=off  pipeline=off
      settings: xl_area=[0, 0, 0, 0, 0, 0, 0]
  DSP48 : xbsIndex_r3/DSP48  pipeline_a=1  use_b=Direct from B Port  pipeline_b=1  pipeline_bcin=1  pipeline_c=on  pipeline_p=on  pipeline_mult=on  pipeline_opmode=on  pipeline_sub=on  pipeline_carryin=on  pipeline_carryinsel=on  use_op=off  use_creg=on  use_pcin=off  use_pcout=off  use_bcout=off  access_rst=off  rst_all=off  rst_a=off  rst_b=off  rst_bcin=off  rst_c=off  rst_mult=off  rst_p=off  rst_ctrl=off  rst_carry_in=off  access_en=off  en_all=off  en_a=off  en_b=off  en_bcin=off  en_c=off  en_mult=off  en_p=off  en_carry_in=off  en_ctrl=off  explicit_period=off  period=1  dbl_ovrd=off  show_param=off  xl_useadderonly=off
      settings: xl_area=[0, 0, 0, 0, 0, 0, 0]  xl_use_area=on
  UDType : xbsIndex_r3/Convert  arith_type="Signed  (2's comp)"  n_bits=16  bin_pt=2  quantization=Truncate  overflow=Wrap  latency=0  explicit_period=off  period=1  dbl_ovrd=off  show_param=off  inserted_by_tool=off  pipeline=off
      settings: xl_area=[0, 0, 0, 0, 0, 0, 0]
  Out1 : Outport
  wires:
  In7/1 -> DSP48/2
  In1/1 -> DSP48/1
  In2/1 -> DSP48/3
  In5/1 -> DSP48/6
  In6/1 -> DSP48/7
  In4/1 -> DSP48/5
  In3/1 -> DSP48/4
  UDType/1 -> Out1/1
  AlignP/1 -> UDType/1
  ConvertP/1 -> AlignP/1
  DSP48/1 -> ConvertP/1

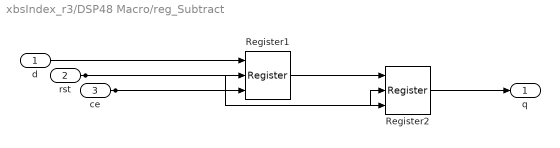
== system xbsIndex_r3/DSP48 Macro/reg_Subtract ==
  d : Inport  Port=1  LatchInput=off
  rst : Inport  Port=2  LatchInput=off
  ce : Inport  Port=3  LatchInput=off
  Register1 : xbsIndex_r3/Register  init=0  reg_only_valid=off  explicit_period=off  period=1  rst=on  en=on  out_en=off  dbl_ovrd=off  show_param=off
      settings: xl_area=[0, 0, 0, 0, 0, 0, 0]
  Register2 : xbsIndex_r3/Register  init=0  reg_only_valid=off  explicit_period=off  period=1  rst=on  en=on  out_en=off  dbl_ovrd=off  show_param=off
      settings: xl_area=[0, 0, 0, 0, 0, 0, 0]
  q : Outport
  wires:
  d/1 -> Register1/1
  rst/1 -> Register1/2, Register2/2
  ce/1 -> Register1/3, Register2/3
  Register1/1 -> Register2/1
  Register2/1 -> q/1

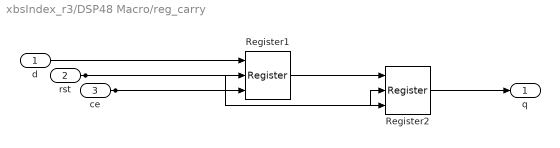
== system xbsIndex_r3/DSP48 Macro/reg_carry ==
  d : Inport  Port=1  LatchInput=off
  rst : Inport  Port=2  LatchInput=off
  ce : Inport  Port=3  LatchInput=off
  Register1 : xbsIndex_r3/Register  init=0  reg_only_valid=off  explicit_period=off  period=1  rst=on  en=on  out_en=off  dbl_ovrd=off  show_param=off
      settings: xl_area=[0, 0, 0, 0, 0, 0, 0]
  Register2 : xbsIndex_r3/Register  init=0  reg_only_valid=off  explicit_period=off  period=1  rst=on  en=on  out_en=off  dbl_ovrd=off  show_param=off
      settings: xl_area=[0, 0, 0, 0, 0, 0, 0]
  q : Outport
  wires:
  d/1 -> Register1/1
  rst/1 -> Register1/2, Register2/2
  ce/1 -> Register1/3, Register2/3
  Register1/1 -> Register2/1
  Register2/1 -> q/1

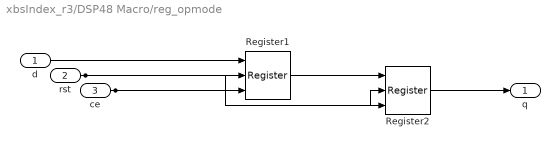
== system xbsIndex_r3/DSP48 Macro/reg_opmode ==
  d : Inport  Port=1  LatchInput=off
  rst : Inport  Port=2  LatchInput=off
  ce : Inport  Port=3  LatchInput=off
  Register1 : xbsIndex_r3/Register  init=0  reg_only_valid=off  explicit_period=off  period=1  rst=on  en=on  out_en=off  dbl_ovrd=off  show_param=off
      settings: xl_area=[0, 0, 0, 0, 0, 0, 0]
  Register2 : xbsIndex_r3/Register  init=0  reg_only_valid=off  explicit_period=off  period=1  rst=on  en=on  out_en=off  dbl_ovrd=off  show_param=off
      settings: xl_area=[0, 0, 0, 0, 0, 0, 0]
  q : Outport
  wires:
  d/1 -> Register1/1
  rst/1 -> Register1/2, Register2/2
  ce/1 -> Register1/3, Register2/3
  Register1/1 -> Register2/1
  Register2/1 -> q/1

== system xbsIndex_r3/PicoBlaze Instruction Display/Write Display ==
  In1 : Inport  Port=1  LatchInput=off
  Trigger : TriggerPort  ZeroCross=off
  S-Function : S-Function  FunctionName=writeDisplay  Parameters=xl_pb_version  mask(Write Display.){sysname=PBDemo_PicoBlaze__Instruction_Display, xl_pb_version=xl_pb_version}
      mask prompts: sysname "System Name"; xl_pb_version "PicoBlaze Version"
      mask help: Write Display. Writes the instruction and program counter to the display block.
  wires:
  In1/1 -> S-Function/1

== system xbsIndex_r3/Single-Step Simulation/Pause  Simulation ==
  din : Inport  Port=1  LatchInput=off
  Pause  Simulation : MATLABFcn  Priority=1000  MATLABFcn=sim_pause(u)  OutputDimensions=0  Output1D=off
  wires:
  din/1 -> Pause  Simulation/1
